simulink model "soal_1"  (R2021b)
settings: Solver=VariableStepAuto  StartTime=0.0  StopTime=10.0  RelTol=1e-3
settings Model: Creator=nnxvnx  LastModifiedBy=Arya

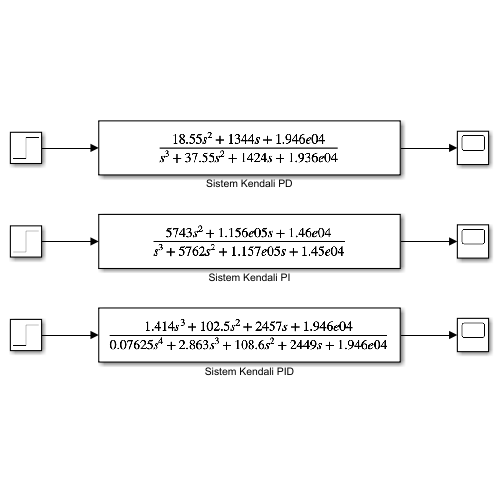
[thumbnail: Simulink's stored preview of the top-level diagram]
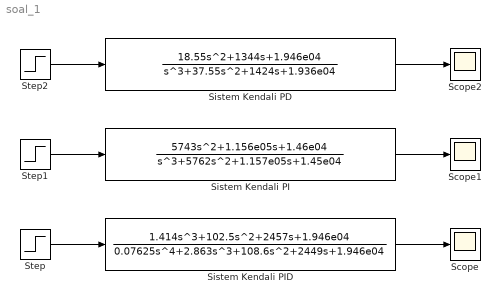
== system soal_1 ==
  Scope : Scope
  Scope1 : Scope
  Scope2 : Scope
  Sistem Kendali PD : TransferFcn  Numerator=[18.55 1344 1.946e04]  Denominator=[1 37.55 1424 1.936e04]
  Sistem Kendali PI : TransferFcn  Numerator=[5743 1.156e05 1.46e04]  Denominator="[1 5762  1.157e05 1.45e04]"
  Sistem Kendali PID : TransferFcn  Numerator=[1.414 102.5 2457 1.946e04]  Denominator=[0.07625 2.863 108.6 2449 1.946e04]
  Step : Step  SampleTime=0
  Step1 : Step  SampleTime=0
  Step2 : Step  SampleTime=0
  wires:
  Step/1 -> Sistem Kendali PID/1
  Sistem Kendali PID/1 -> Scope/1
  Sistem Kendali PI/1 -> Scope1/1
  Step1/1 -> Sistem Kendali PI/1
  Step2/1 -> Sistem Kendali PD/1
  Sistem Kendali PD/1 -> Scope2/1
